simulink library "sp_lib"  (R2019a)
settings: Solver=VariableStepAuto  StartTime=0.0  StopTime=10.0  RelTol=1e-3
undefined symbols (not defined in the file or in its folder): collar_thick, diffuse, flange_len, flange_sep, flange_thick, flange_width, hex_rad, hex_skew, kind_val, leg_rad, lengths, lower_leg_len, shininess, specular, upper_leg_len, X, Y, Z
libraries: sm_lib x26, sm_stewart_platform_lib x10, nesl_utility x7
(part 1 of 2)
settings Model: Creator=mojo  LastModifiedBy=mojo

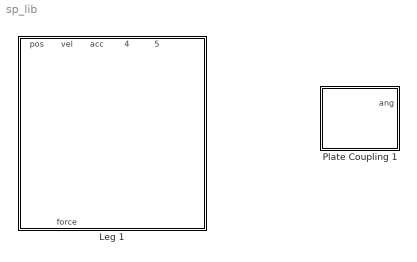
== system sp_lib ==
  Leg 1 : Subsystem  mask(Leg){upper_leg_len=upper_leg_len, lower_leg_len=lower_leg_len, rad=leg_rad, collar_thick=collar_thick, flange_len=flange_len, flange_width=flange_width, flange_thick=flange_thick, asm_offset=lengths(1)}
      mask prompts: upper_leg_len "Upper Leg Length (cm)"; lower_leg_len "Lower Leg Length (cm)"; rad "Radius (cm)"; collar_thick "Collar Thickness (cm)"; flange_len "Flange Length (cm)"; flange_width "Flange Width (cm)"; flange_thick "Flange Thickness (cm)"; asm_offset "Assembly Offset (cm)"
      mask help:
      | Models one of the six identical legs of a Stewart platform manipulator.
      |
      | Each leg is attached to two couplings: one on the base plate of the manipulator and a corresponding one on the platform plate of the manipulator.
      mask Help:
      | A <em>Leg</em> models one of the six identical legs of a Stewart platform manipulator.
      | 
      | Each leg is attached to two couplings: one on the base plate of the manipulator
      | and a corresponding one on the platform plate of the manipulator.
      | 
      | <h3>Components</h3>
      | 
      | A leg is an articulated, non-rigid structure comprising the following parts, listed in
      | top-to-bottom order in the typical orientation of the manipulator.
      | 
      | <ul>
      | <li> Shoulder crosspiece
      | <li> Revolute joint
      | <li> Upper leg
      | <li> Cylindrical knee joint
      | <li> Lower leg
      | <li> Revolute joint
      | <li> Ankle crosspiece
      | </ul>
      | 
      | The two revolute joints adjacent to the two crosspieces each form one half of a universal joint.  The other halves are modeled by revolute joints in the couplings to which the leg is connected.  These connections between legs and couplings could also be modeled by Universal Joint blocks, however, modeling these universal joints with pairs of revolute joints allows for a more detailed model that can display the motion of the universal joint crosspieces.
      | 
      | The leg is divided into upper and lower segments connected through a cylindrical knee joint.  The main portion of each of the two leg segments is modeled as a leg shaft.  Both segments have couplings attached; the upper leg also has a cylindrical extender bar attached.
      | 
      | The revolute primitive of the knee joint is completely passive; it is not actuated.  It is also not sensed.  However, the degree of freedom provided by this primitive is necessary to allow the Stewart platform to move.
      | 
      | The prismatic primitive of the knee joint is force actuated.  The force to be applied to this primitive is provided through a Simulink signal input. This primitive is also sensed: its (linear) position and velocity are available as two Simulink signal outputs.  Typically, a control system will read the current position and velocity and use these to determine a force to be applied to the prismatic primitive of the knee joint to achieve a desired motion of the platform.
      | 
      | Under normal operation, the position of the prismatic primitive of the knee joint should lie within the range [0, L], where L is the length of the lower leg segment.  In the zero configuration of the joint, the upper leg just touches the lower leg, with no gap between them.  A negative joint position will cause the two leg segments to intersect.  Positions exceeding L will cause the extender bar to completely leave the lower leg segment.
      | 
      | <h3>Leg Geometry</h3>
      | 
      | The <em>Geom</em> tab parameters specify the geometry of the main parts of the leg.
      | 
      | <ul>
      | 
      | <li> <b>Upper Leg Length</b> The length of the upper segment of the leg, including the thicknesses of the hexagonal collars but excluding the coupling and extender bar.
      | 
      | <li> <b>Lower Leg Length</b> The length of the lower segment of the leg, including the thicknesses of the hexagonal collars but excluding the coupling.
      | 
      | <li> <b>Radius</b> The radius of the hexagonal cross section of the upper and lower leg segments.
      | 
      | <li> <b>Collar Thickness</b> The thicknesses of the hexagonal collars the upper and lower leg segments.
      | 
      | </ul>
      | 
      | <h3>Flanges</h3>
      | 
      | The <em>Flanges</em> tab parameters specify the geometry of the flanges of the
      | couplings attached to the upper and lower legs.
      | 
      | <ul>
      | 
      | <li> <b>Flange Length</b> The length of the coupling flanges. See <em>Coupling</em> block for details.
      | 
      | <li> <b>Flange Width</b> The width of the coupling flanges. See <em>Coupling</em> block for details.
      | 
      | <li> <b>Flange Thickness</b> The thickness of the coupling flanges. See <em>Coupling</em> block for details.
      | 
      | </ul>
      | 
      | <h3>Assembly</h3>
      | 
      | The <em>Assembly</em> tab parameters specify values to be used during assembly of the Stewart Platform manipulator.
      | 
      | <ul>
      | 
      | <li><b>Assembly Offset</b> The estimated position of the prismatic primitive of the knee joint in the assembled configuration of the Stewart platform manipulator.  This value is used as a suggested joint target for the primitive; it does not have to be exact, and it may not be achieved exactly. Nonetheless, reasonable guesses of this value increase the chances of successful assembly of the manipulator.
      | 
      | </ul>
      | 
      | 
      | <h3>Visualization</h3>
      | 
      | The material properties of a leg's components are all pre-defined and not configurable.
      | 
      | <h3>Ports</h3>
      | 
      | <ul>
      | 
      | <li> <b>base</b> The frame on the leg that should be attached to a coupling on the manipulator's base plate.  This frame is attached to the ankle crosspiece.
      | 
      | <li> <b>platform</b> The frame on the leg that should be attached to a coupling on the manipulator's platform plate.  This frame is attached to the shoulder crosspiece.
      | 
      | <li><b>pos</b> The linear position of the prismatic primitive of the leg's knee joint as a Simulink signal output.  This signal is typically an input to a controller.
      | 
      | <li><b>vel</b> The linear velocity of the prismatic primitive of the leg's knee joint as a Simulink signal output.  This signal is typically an input to a controller.
      | 
      | <li><b>force</b> The force (in N) to be applied to the prismatic primitive of the leg's knee joint as a Simulink signal input.  This signal is typically specified by an output of a controller.  A positive force tends to increase the primitive position.
      | 
      | </ul>
      mask DialogControl ParameterTabVar0 Prompt: Geom
      mask DialogControl ParameterTabVar01 Prompt: Flanges
      mask DialogControl ParameterTabVar012 Prompt: Assembly
      mask Display:
      | image(imread('sm_stewart_platform_leg.png'))
      | color('white')
      | port_label('LConn', 1, 'base')
      | port_label('RConn', 1, 'platform')
      | color('yellow')
      | port_label('Input', 1, 'force')
      | port_label('Output', 1, 'pos')
      | port_label('Output', 2, 'vel')
      | port_label('Output', 3, 'acc')
      | port_label('Output', 4, 'base_ang')
      | port_label('Output', 5, 'plat_ang')
  Plate Coupling 1 : Subsystem  AncestorBlock=sm_stewart_platform_lib/Plate Coupling  mask(Plate Coupling){index=0 + kind_val, hex_rad=hex_rad, hex_skew=hex_skew, flange_width=flange_width, flange_thick=flange_thick, flange_sep=flange_sep, flange_ref_rot=kind_val * 180}
      mask prompts: index "Index (1-6)"; hex_rad "Hexagon Radius (cm)"; hex_skew "Hexagon Skew"; flange_width "Flange Width (cm)"; flange_thick "Flange Thickness (cm)"; flange_sep "Flange Separation (cm)"; flange_ref_rot "Flange Reference Rotation (deg)"
      mask help: Models a coupling with a rigid transform that places it in a specific position and orientation relative to a hexagon plate.
      mask init:
      | % index is in the range [0, 6)
      | sgn = 2 * mod(index + 1, 2) - 1;  % Alternating: +1, -1
      | alpha = (floor((index + 1) / 2) * 120  - 30) * pi/180;
      | theta = (index + sgn * hex_skew) * pi/3;
      | offset = [hex_rad, -(flange_sep + flange_thick) / 2, -flange_width / 2 * sgn] * ...
      |     [0 -sin(theta) +cos(theta); 0 -sin(alpha) +cos(alpha); 0 -cos(alpha) -sin(alpha)];
      mask Help:
      | A <em>Plate Coupling</em> models a coupling with a rigid transform that places it in a specific position and orientation relative to a hexagon plate.
      | 
      | This block serves a specialized role in the modeling of Stewart platform manipulator.  It is used to define the six couplings attached to the lower (base) and upper (platform) hexagon plates of the manipulator.  The plate coupling's initialization function performs the math needed to compute the proper rigid transforms.
      | 
      | <h3>Index</h3>
      | 
      | The <em>Index</em> tab parameters specify the index of the plate coupling.
      | 
      | <ul>
      | 
      | <li> <b>Index</b> The index of the plate coupling, which is an integer in the range [1, 6].  This value indicates which of the six couplings of a hexagonal plate is being defined.  It determines the parameters of the internal rigid transforms that place the coupling at one of the six corners of the skewed hexagon in the proper orientation.
      | 
      | </ul>
      | 
      | <h3>Geometry</h3>
      | 
      | The <em>Geom</em> tab parameters specify the geometry of the plate coupling.
      | 
      | <ul>
      | 
      | <li> <b>Hexagon Radius</b> The radius of the hexagon plate that this plate coupling is attached to.  See <em>Hexagon Plate</em> block for details.
      | 
      | <li> <b>Hexagon Skew</b> The skew factor of the hexagon plate that this plate coupling is attached to.  See <em>Hexagon Plate</em> block for details.
      | 
      | <li> <b>Flange Width</b> The width of the coupling flanges. See <em>Coupling</em> block for details.
      | 
      | <li> <b>Flange Thickness</b> The thickness of the coupling flanges. See <em>Coupling</em> block for details.
      | 
      | <li> <b>Flange Separation</b> The flange separation of the coupling. See <em>Coupling</em> block for details.
      | 
      | <li> <b>Flange Reference Rotation</b> The reference rotation of the coupling.  This value is set to zero for plate couplings attached to the top face of the base plate of the Stewart platform and to 180 degrees for plate couplings attached to the underside of the platform plate.  This aligns the x-axes of all couplings in the upward direction in the zero configuration. See <em>Coupling</em> for details.
      | 
      | </ul>
      | 
      | <h3>Ports</h3>
      | 
      | <ul>
      | 
      | <li> <b>plate</b> The frame of the plate coupling that should be rigidly attached to a frame in the center of the hexagon plate.  The z-axis of this latter frame should be oriented normal to the plane of the plate, and the z-coordinate of its origin should be in the plane of the universal joints attached to the plate.
      | 
      | <li> <b>leg</b> The frame of the plate coupling that should be attached to a leg of the Stewart platform.  Specifically, one of the two crosspieces of the leg is attached to this frame.  The other crosspiece is attached to a corresponding coupling on the other hexagon plate of the manipulator.
      | 
      | </ul>
      mask Display:
      | image(imread('sm_stewart_platform_platecoupling.png'))
      | port_label('LConn', 1, 'plate')
      | port_label('RConn', 1, 'leg')

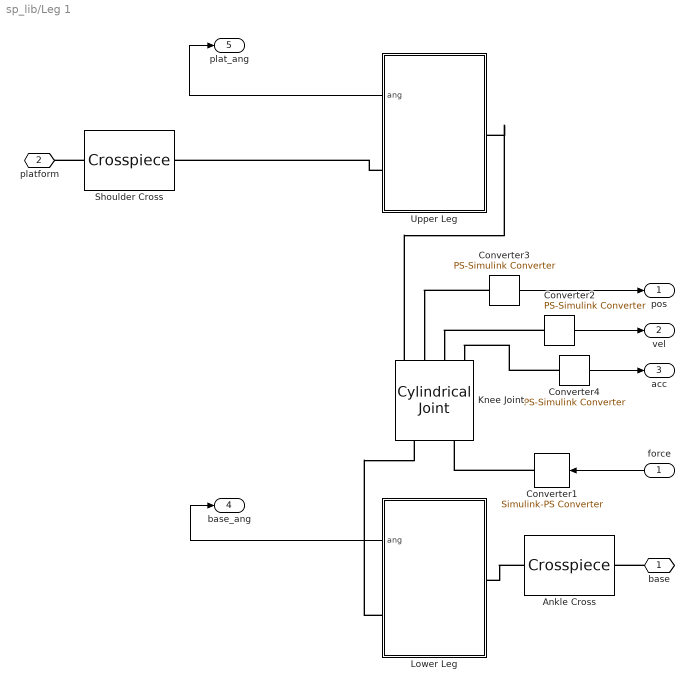
== system sp_lib/Leg 1 ==
  force : Inport
  Ankle Cross : sm_stewart_platform_lib/Crosspiece  arm_len=(rad - flange_thick) * 1.9  arm_rad=rad / 8.0
      settings: SourceProductName=Simscape Multibody  SourceProductBaseCode=MS
  Converter1 : nesl_utility/Simulink-PS Converter  PhysicalDomain=network_engine_domain  SubClassName=ps_input  LeftPortType=input  RightPortType=output  PseudoPeriodic=off  Frequencies=[]  NoiseDistribution=none  NoiseParameters=[]  Unit=N  AffineConversion=off  FilteringAndDerivatives=zero  SimscapeFilterOrder=1  InputFilterTimeConstant=.001  UdotUserProvided=0
  Converter2 : nesl_utility/PS-Simulink Converter  PhysicalDomain=network_engine_domain  SubClassName=ps_output  LeftPortType=input  RightPortType=output  PseudoPeriodic=off  Frequencies=[]  Unit=cm/s  AffineConversion=off
  Converter3 : nesl_utility/PS-Simulink Converter  PhysicalDomain=network_engine_domain  SubClassName=ps_output  LeftPortType=input  RightPortType=output  PseudoPeriodic=off  Frequencies=[]  Unit=cm  AffineConversion=off
  Converter4 : nesl_utility/PS-Simulink Converter  PhysicalDomain=network_engine_domain  SubClassName=ps_output  LeftPortType=input  RightPortType=output  PseudoPeriodic=off  Frequencies=[]  Unit=cm/s/s  AffineConversion=off
  Knee Joint : sm_lib/Joints/Cylindrical Joint  SenseConstraintForce=off  SenseConstraintForceX=off  SenseConstraintForceY=off  SenseConstraintForceZ=off  SenseConstraintTorque=off  SenseConstraintTorqueX=off  SenseConstraintTorqueY=off  SenseConstraintTorqueZ=off  SenseTotalForce=off  SenseTotalForceX=off  SenseTotalForceY=off  SenseTotalForceZ=off  SenseTotalTorque=off  SenseTotalTorqueX=off  SenseTotalTorqueY=off  SenseTotalTorqueZ=off  CompositeWrenchDir=FollowerOnBase  CompositeWrenchFrame=BaseFrame  PzEquilibriumPosition=0  PzEquilibriumPositionUnits=m  PzSpringStiffness=0  PzSpringStiffnessUnits=N/m  PzDampingCoefficient=0  PzDampingCoefficientUnits=N/(m/s)  PzTorqueActuationMode=InputTorque  PzMotionActuationMode=ComputedMotion  PzSensePosition=on  PzSenseVelocity=on  PzSenseAcceleration=on  PzSenseTorqueForce=off  PzSenseLowerLimitTorqueForce=off  PzSenseUpperLimitTorqueForce=off  PzLowerLimitSpecify=off  PzLowerLimitBound=-1  PzLowerLimitBoundUnits=m  PzLowerLimitStiffness=1e6  PzLowerLimitStiffnessUnits=N/m  PzLowerLimitDamping=1e3  PzLowerLimitDampingUnits=N/(m/s)  PzLowerLimitTransitionRegionWidth=1e-4  PzLowerLimitTransitionRegionWidthUnits=m  PzUpperLimitSpecify=off  PzUpperLimitBound=1  PzUpperLimitBoundUnits=m  PzUpperLimitStiffness=1e6  PzUpperLimitStiffnessUnits=N/m  PzUpperLimitDamping=1e3  PzUpperLimitDampingUnits=N/(m/s)  PzUpperLimitTransitionRegionWidth=1e-4  PzUpperLimitTransitionRegionWidthUnits=m  PzPositionTargetSpecify=on  PzPositionTargetPriority=High  PzPositionTargetValue=asm_offset  PzPositionTargetValueUnits=cm  PzVelocityTargetSpecify=off  PzVelocityTargetPriority=High  PzVelocityTargetValue=0  PzVelocityTargetValueUnits=m/s  RzEquilibriumPosition=0  RzEquilibriumPositionUnits=rad  RzSpringStiffness=0  RzSpringStiffnessUnits=N*m/rad  RzDampingCoefficient=0  RzDampingCoefficientUnits=N*m/(rad/s)  RzTorqueActuationMode=NoTorque  RzMotionActuationMode=ComputedMotion  RzSensePosition=off  RzSenseVelocity=off  RzSenseAcceleration=off  RzSenseTorqueForce=off  RzSenseLowerLimitTorqueForce=off  RzSenseUpperLimitTorqueForce=off  RzLowerLimitSpecify=off  RzLowerLimitBound=-90  RzLowerLimitBoundUnits=deg  RzLowerLimitStiffness=1e4  RzLowerLimitStiffnessUnits=N*m/deg  RzLowerLimitDamping=10  RzLowerLimitDampingUnits=N*m/(deg/s)  RzLowerLimitTransitionRegionWidth=0.1  RzLowerLimitTransitionRegionWidthUnits=deg  RzUpperLimitSpecify=off  RzUpperLimitBound=90  RzUpperLimitBoundUnits=deg  RzUpperLimitStiffness=1e4  RzUpperLimitStiffnessUnits=N*m/deg  RzUpperLimitDamping=10  RzUpperLimitDampingUnits=N*m/(deg/s)  RzUpperLimitTransitionRegionWidth=0.1  RzUpperLimitTransitionRegionWidthUnits=deg  RzPositionTargetSpecify=off  RzPositionTargetPriority=High  RzPositionTargetValue=0  RzPositionTargetValueUnits=rad  RzVelocityTargetSpecify=off  RzVelocityTargetPriority=High  RzVelocityTargetValue=0  RzVelocityTargetValueUnits=rad/s
  Lower Leg : Subsystem
      mask Display:
      | image(imread('sm_stewart_platform_lowerleg.png'))
      | color('white')
      | port_label('LConn', 1, 'lower')
      | port_label('RConn', 1, 'upper')
      | port_label('Output', 1, 'ang')
  Shoulder Cross : sm_stewart_platform_lib/Crosspiece  arm_len=(rad - flange_thick) * 1.9  arm_rad=rad / 8.0
      settings: SourceProductName=Simscape Multibody  SourceProductBaseCode=MS
  Upper Leg : Subsystem
      mask Display:
      | image(imread('sm_stewart_platform_upperleg.png'))
      | color('white')
      | port_label('LConn', 1, 'lower')
      | port_label('RConn', 1, 'upper')
      | port_label('Output', 1, 'ang')
  base : PMIOPort  Side=Left
  platform : PMIOPort  Port=2  Side=Right
  pos : Outport
  vel : Outport  Port=2
  acc : Outport  Port=3
  base_ang : Outport  Port=4
  plat_ang : Outport  Port=5
  wires:
  Converter3/1 -> pos/1
  Converter2/1 -> vel/1
  force/1 -> Converter1/1
  Converter4/1 -> acc/1
  Lower Leg/1(ang) -> base_ang/1
  Upper Leg/1(ang) -> plat_ang/1
  connections:
  Converter3/LConn1 -- Knee Joint/RConn2
  Converter2/LConn1 -- Knee Joint/RConn3
  Converter1/RConn1 -- Knee Joint/LConn2
  Knee Joint/RConn1 -- Upper Leg/LConn1
  Lower Leg/RConn1 -- Knee Joint/LConn1
  base/RConn1 -- Ankle Cross/LConn1
  Ankle Cross/RConn1 -- Lower Leg/LConn1
  Upper Leg/RConn1 -- Shoulder Cross/LConn1
  Shoulder Cross/RConn1 -- platform/RConn1
  Converter4/LConn1 -- Knee Joint/RConn4

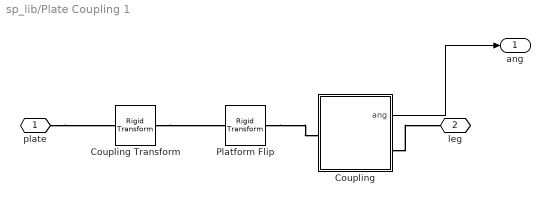
== system sp_lib/Plate Coupling 1 ==
  Coupling : Subsystem  AncestorBlock=sm_stewart_platform_lib/Coupling  mask(Coupling){flange_sep=flange_sep, flange_len=flange_len, flange_width=flange_width, flange_thick=flange_thick, ref_rot=flange_ref_rot, diffuse=diffuse, specular=specular, shininess=shininess}
      mask prompts: flange_sep "Flange Separation (cm)"; flange_len "Flange Length (cm)"; flange_width "Flange Width (cm)"; flange_thick "Flange Thickness (cm)"; ref_rot "Reference Rotation (deg)"; diffuse "Diffuse (rgba)"; specular "Specular (rgba)"; shininess "Shininess (0-128)"
      mask help: Models a pair of parallel flanges with a revolute joint between them.
      mask Help:
      | A <em>Coupling</em> models a pair of parallel flanges with a revolute joint between them.  The axis of the revolute joint is normal to the planes of the flanges.
      | 
      | In a Stewart platform, couplings attached to the base, legs, and platform are used to anchor the arms of the universal joint crosspieces.
      | 
      | <h3>Geometry</h3>
      | 
      | The <em>Geom</em> tab parameters specify the geometry of the coupling.
      | 
      | <ul>
      | 
      | <li> <b>Flange Separation</b> The distance between the origins of the reference frames of the two flanges.  These are located within the interiors of the flanges; the distance between the facing surfaces of the flanges is one flange thickness less than this amount.
      | 
      | <li> <b>Length</b> The length of the flanges.  See <em>Flange</em> block for details.
      | 
      | <li> <b>Width</b> The width of the flanges.  See <em>Flange</em> block for details.
      | 
      | <li> <b>Thickness</b> The thickness of the flanges.  See <em>Flange</em> block for details.
      | 
      | <li> <b>Reference Rotation</b> A value specifying the zero point for the coupling's revolute joint.  A value of zero makes the zero configuration the one in which the x-axis of the <em>rot</em> frame is directed toward the curved end caps of the flanges.  A value of 180 degrees makes the zero configuration the one in which the x-axis of the <em>rot</em> frame is directed away from the curved end caps of the flanges.
      | 
      | </ul>
      | 
      | <h3>Visualization</h3>
      | 
      | The <em>Graphics</em> tab parameters specify the visualization aspects of the coupling.  Both flanges of the coupling have the same visual properties.
      | 
      | <ul>
      | 
      | <li> <b>Diffuse</b> The diffuse color of the coupling.  This is an RGB 3-vector or an RGBA 4-vector with all components in the range [0, 1].
      | 
      | <li> <b>Specular</b> The specular color of the coupling.  This is an RGB 3-vector or an RGBA 4-vector with all components in the range [0, 1].
      | 
      | <li> <b>Shininess</b> The shininess of the coupling.  This is a scalar value in the range [0, 128].
      | 
      | </ul>
      | 
      | 
      | <h3>Ports</h3>
      | 
      | <ul>
      | 
      | <li> <b>ref</b> The reference frame of the coupling.  This is also the base frame of the coupling's revolute joint.  The origin is at the midpoint of the line segment joining the reference frame origins of the two flanges.  The z-axis is normal to the planes of the flanges.  The x-axis direction depends on the setting of <em>Reference Roation</em> (see above).
      | 
      | <li> <b>rot</b> The rotated frame of the coupling.  This is also the follower frame of the coupling's revolute joint.  The origin is at the midpoint of the line segment joining the reference frame origins of the two flanges.  The z-axis is normal to the planes of the flanges.  The x-axis direction depends on the setting of <em>Reference Roation</em> (see above) and on the revolute joint's position.
      | 
      | </ul>
      | 
      | Typically, a coupling is rigidly attached to a host body through its <em>ref</em> port.  The body attached to its <em>rot</em> port can rotate about the coupling axis with respect to the host body.
      mask Display:
      | image(imread('sm_stewart_platform_coupling.png'))
      | color('white')
      | port_label('LConn', 1, 'ref')
      | port_label('RConn', 1, 'rot')
  Coupling Transform : sm_lib/Frames and Transforms/Rigid Transform  TranslationMethod=Cartesian  TranslationStandardOffset=0  TranslationLengthUnit=cm  TranslationStandardAxis=+Z  TranslationCartesianOffset=offset  TranslationROffset=0  TranslationROffsetUnits=m  TranslationZOffset=0  TranslationZOffsetUnits=m  TranslationThetaOffset=0  TranslationThetaOffsetUnits=deg  RotationMethod=StandardAxis  RotationAngleUnits=rad  RotationStandardAxis=+X  RotationAngle=alpha  RotationArbitraryAxis=[0 0 1]  FollAlignAxisA=+X  BaseAlignAxisA=+Y  FollAlignAxisB=+Y  BaseAlignAxisB=+Z  RotationSequenceAxes=FollowerAxes  RotationSequence=XYX  RotationSequenceAngles=[0 0 0]  RotationSequenceAnglesUnits=deg  RotationMatrix=[1 0 0; 0 1 0; 0 0 1]
  Platform Flip : sm_lib/Frames and Transforms/Rigid Transform  TranslationMethod=None  TranslationStandardOffset=0  TranslationLengthUnit=m  TranslationStandardAxis=+Z  TranslationCartesianOffset=[0 0 0]  TranslationROffset=0  TranslationROffsetUnits=m  TranslationZOffset=0  TranslationZOffsetUnits=m  TranslationThetaOffset=0  TranslationThetaOffsetUnits=deg  RotationMethod=StandardAxis  RotationAngleUnits=deg  RotationStandardAxis=+Z  RotationAngle=kind_val * 180  RotationArbitraryAxis=[0 0 1]  FollAlignAxisA=+X  BaseAlignAxisA=+Y  FollAlignAxisB=+Y  BaseAlignAxisB=+Z  RotationSequenceAxes=FollowerAxes  RotationSequence=XYX  RotationSequenceAngles=[0 0 0]  RotationSequenceAnglesUnits=deg  RotationMatrix=[1 0 0; 0 1 0; 0 0 1]
  plate : PMIOPort  Side=Left
  leg : PMIOPort  Port=2  Side=Right
  ang : Outport
  wires:
  Coupling/1(ang) -> ang/1
  connections:
  plate/RConn1 -- Coupling Transform/LConn1
  Coupling Transform/RConn1 -- Platform Flip/LConn1
  Platform Flip/RConn1 -- Coupling/LConn1
  Coupling/RConn1 -- leg/RConn1

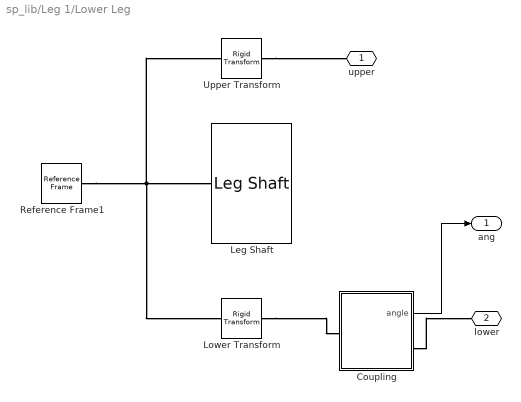
== system sp_lib/Leg 1/Lower Leg ==
  Coupling : Subsystem  AncestorBlock=sm_stewart_platform_lib/Coupling  mask(Coupling){flange_sep=2 * rad * cos(pi/6) - flange_thick, flange_len=flange_len, flange_width=flange_width, flange_thick=flange_thick, ref_rot=180, diffuse=[.5 .5 .6], specular=[.8 .8 1], shininess=100}
      mask prompts: flange_sep "Flange Separation (cm)"; flange_len "Flange Length (cm)"; flange_width "Flange Width (cm)"; flange_thick "Flange Thickness (cm)"; ref_rot "Reference Rotation (deg)"; diffuse "Diffuse (rgba)"; specular "Specular (rgba)"; shininess "Shininess (0-128)"
      mask help: Models a pair of parallel flanges with a revolute joint between them.
      mask Help:
      | A <em>Coupling</em> models a pair of parallel flanges with a revolute joint between them.  The axis of the revolute joint is normal to the planes of the flanges.
      | 
      | In a Stewart platform, couplings attached to the base, legs, and platform are used to anchor the arms of the universal joint crosspieces.
      | 
      | <h3>Geometry</h3>
      | 
      | The <em>Geom</em> tab parameters specify the geometry of the coupling.
      | 
      | <ul>
      | 
      | <li> <b>Flange Separation</b> The distance between the origins of the reference frames of the two flanges.  These are located within the interiors of the flanges; the distance between the facing surfaces of the flanges is one flange thickness less than this amount.
      | 
      | <li> <b>Length</b> The length of the flanges.  See <em>Flange</em> block for details.
      | 
      | <li> <b>Width</b> The width of the flanges.  See <em>Flange</em> block for details.
      | 
      | <li> <b>Thickness</b> The thickness of the flanges.  See <em>Flange</em> block for details.
      | 
      | <li> <b>Reference Rotation</b> A value specifying the zero point for the coupling's revolute joint.  A value of zero makes the zero configuration the one in which the x-axis of the <em>rot</em> frame is directed toward the curved end caps of the flanges.  A value of 180 degrees makes the zero configuration the one in which the x-axis of the <em>rot</em> frame is directed away from the curved end caps of the flanges.
      | 
      | </ul>
      | 
      | <h3>Visualization</h3>
      | 
      | The <em>Graphics</em> tab parameters specify the visualization aspects of the coupling.  Both flanges of the coupling have the same visual properties.
      | 
      | <ul>
      | 
      | <li> <b>Diffuse</b> The diffuse color of the coupling.  This is an RGB 3-vector or an RGBA 4-vector with all components in the range [0, 1].
      | 
      | <li> <b>Specular</b> The specular color of the coupling.  This is an RGB 3-vector or an RGBA 4-vector with all components in the range [0, 1].
      | 
      | <li> <b>Shininess</b> The shininess of the coupling.  This is a scalar value in the range [0, 128].
      | 
      | </ul>
      | 
      | 
      | <h3>Ports</h3>
      | 
      | <ul>
      | 
      | <li> <b>ref</b> The reference frame of the coupling.  This is also the base frame of the coupling's revolute joint.  The origin is at the midpoint of the line segment joining the reference frame origins of the two flanges.  The z-axis is normal to the planes of the flanges.  The x-axis direction depends on the setting of <em>Reference Roation</em> (see above).
      | 
      | <li> <b>rot</b> The rotated frame of the coupling.  This is also the follower frame of the coupling's revolute joint.  The origin is at the midpoint of the line segment joining the reference frame origins of the two flanges.  The z-axis is normal to the planes of the flanges.  The x-axis direction depends on the setting of <em>Reference Roation</em> (see above) and on the revolute joint's position.
      | 
      | </ul>
      | 
      | Typically, a coupling is rigidly attached to a host body through its <em>ref</em> port.  The body attached to its <em>rot</em> port can rotate about the coupling axis with respect to the host body.
      mask Display:
      | image(imread('sm_stewart_platform_coupling.png'))
      | color('white')
      | port_label('LConn', 1, 'ref')
      | port_label('RConn', 1, 'rot')
  Leg Shaft : sm_stewart_platform_lib/Leg Shaft  length=lower_leg_len  rad=rad  collar_thick=collar_thick  color=[0 0 0.6]
      settings: SourceProductName=Simscape Multibody  SourceProductBaseCode=MS
  Lower Transform : sm_lib/Frames and Transforms/Rigid Transform  TranslationMethod=StandardAxis  TranslationStandardOffset=lower_leg_len / 2 + flange_len  TranslationLengthUnit=cm  TranslationStandardAxis=-Z  TranslationCartesianOffset=[0 0 0]  TranslationROffset=0  TranslationROffsetUnits=m  TranslationZOffset=0  TranslationZOffsetUnits=m  TranslationThetaOffset=0  TranslationThetaOffsetUnits=deg  RotationMethod=AlignedAxes  RotationAngleUnits=deg  RotationStandardAxis=+Z  RotationAngle=0  RotationArbitraryAxis=[0 0 1]  FollAlignAxisA=+Z  BaseAlignAxisA=+X  FollAlignAxisB=+X  BaseAlignAxisB=-Z  RotationSequenceAxes=FollowerAxes  RotationSequence=XYX  RotationSequenceAngles=[0 0 0]  RotationSequenceAnglesUnits=deg  RotationMatrix=[1 0 0; 0 1 0; 0 0 1]
  Reference Frame1 : sm_lib/Frames and Transforms/Reference Frame
  Upper Transform : sm_lib/Frames and Transforms/Rigid Transform  TranslationMethod=StandardAxis  TranslationStandardOffset=lower_leg_len / 2  TranslationLengthUnit=cm  TranslationStandardAxis=+Z  TranslationCartesianOffset=[0 0 0]  TranslationROffset=0  TranslationROffsetUnits=m  TranslationZOffset=0  TranslationZOffsetUnits=m  TranslationThetaOffset=0  TranslationThetaOffsetUnits=deg  RotationMethod=None  RotationAngleUnits=deg  RotationStandardAxis=+Z  RotationAngle=0  RotationArbitraryAxis=[0 0 1]  FollAlignAxisA=+X  BaseAlignAxisA=+Y  FollAlignAxisB=+Y  BaseAlignAxisB=+Z  RotationSequenceAxes=FollowerAxes  RotationSequence=XYX  RotationSequenceAngles=[0 0 0]  RotationSequenceAnglesUnits=deg  RotationMatrix=[1 0 0; 0 1 0; 0 0 1]
  upper : PMIOPort  Side=Right
  lower : PMIOPort  Port=2  Side=Left
  ang : Outport
  wires:
  Coupling/1(angle) -> ang/1
  connections:
  Reference Frame1/RConn1 -- Upper Transform/LConn1 -- Lower Transform/LConn1 -- Leg Shaft/LConn1
  Coupling/RConn1 -- lower/RConn1
  Upper Transform/RConn1 -- upper/RConn1
  Lower Transform/RConn1 -- Coupling/LConn1

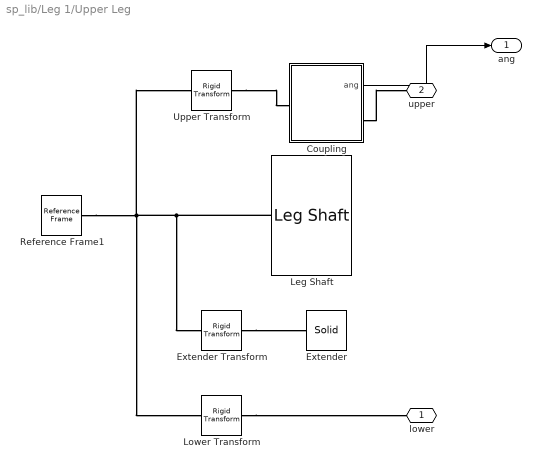
== system sp_lib/Leg 1/Upper Leg ==
  Coupling : Subsystem  AncestorBlock=sm_stewart_platform_lib/Coupling  mask(Coupling){flange_sep=2 * rad * cos(pi/6) - flange_thick, flange_len=flange_len, flange_width=flange_width, flange_thick=flange_thick, ref_rot=0, diffuse=[.5 .5 .6], specular=[.8 .8 1], shininess=100}
      mask prompts: flange_sep "Flange Separation (cm)"; flange_len "Flange Length (cm)"; flange_width "Flange Width (cm)"; flange_thick "Flange Thickness (cm)"; ref_rot "Reference Rotation (deg)"; diffuse "Diffuse (rgba)"; specular "Specular (rgba)"; shininess "Shininess (0-128)"
      mask help: Models a pair of parallel flanges with a revolute joint between them.
      mask Help:
      | A <em>Coupling</em> models a pair of parallel flanges with a revolute joint between them.  The axis of the revolute joint is normal to the planes of the flanges.
      | 
      | In a Stewart platform, couplings attached to the base, legs, and platform are used to anchor the arms of the universal joint crosspieces.
      | 
      | <h3>Geometry</h3>
      | 
      | The <em>Geom</em> tab parameters specify the geometry of the coupling.
      | 
      | <ul>
      | 
      | <li> <b>Flange Separation</b> The distance between the origins of the reference frames of the two flanges.  These are located within the interiors of the flanges; the distance between the facing surfaces of the flanges is one flange thickness less than this amount.
      | 
      | <li> <b>Length</b> The length of the flanges.  See <em>Flange</em> block for details.
      | 
      | <li> <b>Width</b> The width of the flanges.  See <em>Flange</em> block for details.
      | 
      | <li> <b>Thickness</b> The thickness of the flanges.  See <em>Flange</em> block for details.
      | 
      | <li> <b>Reference Rotation</b> A value specifying the zero point for the coupling's revolute joint.  A value of zero makes the zero configuration the one in which the x-axis of the <em>rot</em> frame is directed toward the curved end caps of the flanges.  A value of 180 degrees makes the zero configuration the one in which the x-axis of the <em>rot</em> frame is directed away from the curved end caps of the flanges.
      | 
      | </ul>
      | 
      | <h3>Visualization</h3>
      | 
      | The <em>Graphics</em> tab parameters specify the visualization aspects of the coupling.  Both flanges of the coupling have the same visual properties.
      | 
      | <ul>
      | 
      | <li> <b>Diffuse</b> The diffuse color of the coupling.  This is an RGB 3-vector or an RGBA 4-vector with all components in the range [0, 1].
      | 
      | <li> <b>Specular</b> The specular color of the coupling.  This is an RGB 3-vector or an RGBA 4-vector with all components in the range [0, 1].
      | 
      | <li> <b>Shininess</b> The shininess of the coupling.  This is a scalar value in the range [0, 128].
      | 
      | </ul>
      | 
      | 
      | <h3>Ports</h3>
      | 
      | <ul>
      | 
      | <li> <b>ref</b> The reference frame of the coupling.  This is also the base frame of the coupling's revolute joint.  The origin is at the midpoint of the line segment joining the reference frame origins of the two flanges.  The z-axis is normal to the planes of the flanges.  The x-axis direction depends on the setting of <em>Reference Roation</em> (see above).
      | 
      | <li> <b>rot</b> The rotated frame of the coupling.  This is also the follower frame of the coupling's revolute joint.  The origin is at the midpoint of the line segment joining the reference frame origins of the two flanges.  The z-axis is normal to the planes of the flanges.  The x-axis direction depends on the setting of <em>Reference Roation</em> (see above) and on the revolute joint's position.
      | 
      | </ul>
      | 
      | Typically, a coupling is rigidly attached to a host body through its <em>ref</em> port.  The body attached to its <em>rot</em> port can rotate about the coupling axis with respect to the host body.
      mask Display:
      | image(imread('sm_stewart_platform_coupling.png'))
      | color('white')
      | port_label('LConn', 1, 'ref')
      | port_label('RConn', 1, 'rot')
  Extender : sm_lib/Body Elements/Solid  InertiaType=CalculateFromGeometry  Mass=1  MassUnits=kg  CenterOfMass=[0 0 0]  CenterOfMassUnits=m  MomentsOfInertia=[1 1 1]  MomentsOfInertiaUnits=kg*m^2  ProductsOfInertia=[0 0 0]  ProductsOfInertiaUnits=kg*m^2  BasedOnType=Density  Density=g_density  DensityUnits=g/cm^3  DoExposeReferenceFrame=on  SerializedFrames=<Frames/>  GraphicType=FromGeometry  MarkerShape=Sphere  MarkerSize=1  MarkerSizeUnits=m  GraphicVisPropType=AdvancedVisualProperties  GraphicDiffuseColor=[.5 .5 .6]  GraphicSpecularColor=[.8 .8 1]  GraphicAmbientColor=[ 0.1 0.1 0.1 ]  GraphicEmissiveColor=[ 0 0 0]  GraphicShininess=100  GraphicOpacity=1  GeometryShape=Cylinder  RectangleSize=[1 1]  RectangleSizeUnits=m  BrickDimensions=[1 1 1]  BrickDimensionUnits=m  CylinderRadius=rad / 2  CylinderRadiusUnits=cm  CylinderLength=lower_leg_len  CylinderLengthUnits=cm  SphereRadius=1  SphereRadiusUnits=m  EllipsoidRadii=[1 1 1]  EllipsoidRadiiUnits=m  ExtrusionCrossSection=[1 1; -1 1; -1 -1; 1 -1]  ExtrusionCrossSectionUnits=m  ExtrusionLength=lower_leg_len  ExtrusionLengthUnits=cm  PolygonNumSides=6  PolygonOuterRadius=rad / 2  PolygonOuterRadiusUnits=cm  ExtGeomFileType=STEP  ExtGeomFileUnits=m  RevolutionCrossSection=[1 1; 1 -1; 2 -1; 2 1]  RevolutionCrossSectionUnits=m  RevolutionExtent=Full  RevolutionAngle=180  RevolutionAngleUnits=deg
  Extender Transform : sm_lib/Frames and Transforms/Rigid Transform  TranslationMethod=StandardAxis  TranslationStandardOffset=(upper_leg_len + lower_leg_len) / 2  TranslationLengthUnit=cm  TranslationStandardAxis=-Z  TranslationCartesianOffset=[0 0 0]  TranslationROffset=0  TranslationROffsetUnits=m  TranslationZOffset=0  TranslationZOffsetUnits=m  TranslationThetaOffset=0  TranslationThetaOffsetUnits=deg  RotationMethod=StandardAxis  RotationAngleUnits=deg  RotationStandardAxis=+Z  RotationAngle=30  RotationArbitraryAxis=[0 0 1]  FollAlignAxisA=+X  BaseAlignAxisA=+Y  FollAlignAxisB=+Y  BaseAlignAxisB=+Z  RotationSequenceAxes=FollowerAxes  RotationSequence=XYX  RotationSequenceAngles=[0 0 0]  RotationSequenceAnglesUnits=deg  RotationMatrix=[1 0 0; 0 1 0; 0 0 1]
  Leg Shaft : sm_stewart_platform_lib/Leg Shaft  length=upper_leg_len  rad=rad  collar_thick=collar_thick  color=[0.6 0 0]
      settings: SourceProductName=Simscape Multibody  SourceProductBaseCode=MS
  Lower Transform : sm_lib/Frames and Transforms/Rigid Transform  TranslationMethod=StandardAxis  TranslationStandardOffset=upper_leg_len / 2  TranslationLengthUnit=cm  TranslationStandardAxis=-Z  TranslationCartesianOffset=[0 0 0]  TranslationROffset=0  TranslationROffsetUnits=m  TranslationZOffset=0  TranslationZOffsetUnits=m  TranslationThetaOffset=0  TranslationThetaOffsetUnits=deg  RotationMethod=None  RotationAngleUnits=deg  RotationStandardAxis=+Z  RotationAngle=0  RotationArbitraryAxis=[0 0 1]  FollAlignAxisA=+X  BaseAlignAxisA=+Y  FollAlignAxisB=+Y  BaseAlignAxisB=+Z  RotationSequenceAxes=FollowerAxes  RotationSequence=XYX  RotationSequenceAngles=[0 0 0]  RotationSequenceAnglesUnits=deg  RotationMatrix=[1 0 0; 0 1 0; 0 0 1]
  Reference Frame1 : sm_lib/Frames and Transforms/Reference Frame
  Upper Transform : sm_lib/Frames and Transforms/Rigid Transform  TranslationMethod=StandardAxis  TranslationStandardOffset=upper_leg_len / 2 + flange_len  TranslationLengthUnit=cm  TranslationStandardAxis=+Z  TranslationCartesianOffset=[0 0 0]  TranslationROffset=0  TranslationROffsetUnits=m  TranslationZOffset=0  TranslationZOffsetUnits=m  TranslationThetaOffset=0  TranslationThetaOffsetUnits=deg  RotationMethod=AlignedAxes  RotationAngleUnits=deg  RotationStandardAxis=+Z  RotationAngle=0  RotationArbitraryAxis=[0 0 1]  FollAlignAxisA=+Z  BaseAlignAxisA=-X  FollAlignAxisB=+X  BaseAlignAxisB=+Z  RotationSequenceAxes=FollowerAxes  RotationSequence=XYX  RotationSequenceAngles=[0 0 0]  RotationSequenceAnglesUnits=deg  RotationMatrix=[1 0 0; 0 1 0; 0 0 1]
  lower : PMIOPort  Side=Left
  upper : PMIOPort  Port=2  Side=Right
  ang : Outport
  wires:
  Coupling/1(ang) -> ang/1
  connections:
  Upper Transform/RConn1 -- Coupling/LConn1
  Lower Transform/RConn1 -- lower/RConn1
  Coupling/RConn1 -- upper/RConn1
  Leg Shaft/LConn1 -- Reference Frame1/RConn1 -- Upper Transform/LConn1 -- Lower Transform/LConn1 -- Extender Transform/LConn1
  Extender Transform/RConn1 -- Extender/RConn1

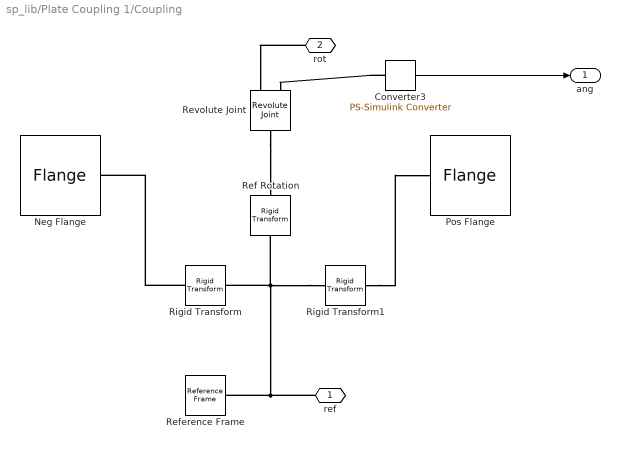
== system sp_lib/Plate Coupling 1/Coupling ==
  Converter3 : nesl_utility/PS-Simulink Converter  PhysicalDomain=network_engine_domain  SubClassName=ps_output  LeftPortType=input  RightPortType=output  PseudoPeriodic=off  Frequencies=[]  Unit=deg  AffineConversion=off
  Neg Flange : sm_stewart_platform_lib/Flange  len=flange_len  width=flange_width  thick=flange_thick  diffuse=diffuse  specular=specular  shininess=shininess
      settings: SourceProductName=Simscape Multibody  SourceProductBaseCode=MS
  Pos Flange : sm_stewart_platform_lib/Flange  len=flange_len  width=flange_width  thick=flange_thick  diffuse=diffuse  specular=specular  shininess=shininess
      settings: SourceProductName=Simscape Multibody  SourceProductBaseCode=MS
  Ref Rotation : sm_lib/Frames and Transforms/Rigid Transform  TranslationMethod=None  TranslationStandardOffset=0  TranslationLengthUnit=m  TranslationStandardAxis=+Z  TranslationCartesianOffset=[0 0 0]  TranslationROffset=0  TranslationROffsetUnits=m  TranslationZOffset=0  TranslationZOffsetUnits=m  TranslationThetaOffset=0  TranslationThetaOffsetUnits=deg  RotationMethod=StandardAxis  RotationAngleUnits=deg  RotationStandardAxis=+Z  RotationAngle=ref_rot  RotationArbitraryAxis=[0 0 1]  FollAlignAxisA=+X  BaseAlignAxisA=+Y  FollAlignAxisB=+Y  BaseAlignAxisB=+Z  RotationSequenceAxes=FollowerAxes  RotationSequence=XYX  RotationSequenceAngles=[0 0 0]  RotationSequenceAnglesUnits=deg  RotationMatrix=[1 0 0; 0 1 0; 0 0 1]
  Reference Frame : sm_lib/Frames and Transforms/Reference Frame
  Revolute Joint : sm_lib/Joints/Revolute Joint  SenseConstraintForce=off  SenseConstraintForceX=off  SenseConstraintForceY=off  SenseConstraintForceZ=off  SenseConstraintTorque=off  SenseConstraintTorqueX=off  SenseConstraintTorqueY=off  SenseConstraintTorqueZ=off  SenseTotalForce=off  SenseTotalForceX=off  SenseTotalForceY=off  SenseTotalForceZ=off  SenseTotalTorque=off  SenseTotalTorqueX=off  SenseTotalTorqueY=off  SenseTotalTorqueZ=off  CompositeWrenchDir=FollowerOnBase  CompositeWrenchFrame=BaseFrame  EquilibriumPosition=0  EquilibriumPositionUnits=rad  SpringStiffness=0  SpringStiffnessUnits=N*m/rad  DampingCoefficient=0  DampingCoefficientUnits=N*m/(rad/s)  TorqueActuationMode=NoTorque  MotionActuationMode=ComputedMotion  SensePosition=on  SenseVelocity=off  SenseAcceleration=off  SenseTorqueForce=off  SenseLowerLimitTorqueForce=off  SenseUpperLimitTorqueForce=off  LowerLimitSpecify=off  LowerLimitBound=-90  LowerLimitBoundUnits=deg  LowerLimitStiffness=1e4  LowerLimitStiffnessUnits=N*m/deg  LowerLimitDamping=10  LowerLimitDampingUnits=N*m/(deg/s)  LowerLimitTransitionRegionWidth=0.1  LowerLimitTransitionRegionWidthUnits=deg  UpperLimitSpecify=off  UpperLimitBound=90  UpperLimitBoundUnits=deg  UpperLimitStiffness=1e4  UpperLimitStiffnessUnits=N*m/deg  UpperLimitDamping=10  UpperLimitDampingUnits=N*m/(deg/s)  UpperLimitTransitionRegionWidth=0.1  UpperLimitTransitionRegionWidthUnits=deg  PositionTargetSpecify=off  PositionTargetPriority=High  PositionTargetValue=0  PositionTargetValueUnits=rad  VelocityTargetSpecify=off  VelocityTargetPriority=High  VelocityTargetValue=0  VelocityTargetValueUnits=rad/s
  Rigid Transform : sm_lib/Frames and Transforms/Rigid Transform  TranslationMethod=StandardAxis  TranslationStandardOffset=flange_sep / 2  TranslationLengthUnit=cm  TranslationStandardAxis=-Z  TranslationCartesianOffset=[0 0 0]  TranslationROffset=0  TranslationROffsetUnits=m  TranslationZOffset=0  TranslationZOffsetUnits=m  TranslationThetaOffset=0  TranslationThetaOffsetUnits=deg  RotationMethod=None  RotationAngleUnits=deg  RotationStandardAxis=+Z  RotationAngle=0  RotationArbitraryAxis=[0 0 1]  FollAlignAxisA=+X  BaseAlignAxisA=+Y  FollAlignAxisB=+Y  BaseAlignAxisB=+Z  RotationSequenceAxes=FollowerAxes  RotationSequence=XYX  RotationSequenceAngles=[0 0 0]  RotationSequenceAnglesUnits=deg  RotationMatrix=[1 0 0; 0 1 0; 0 0 1]
  Rigid Transform1 : sm_lib/Frames and Transforms/Rigid Transform  TranslationMethod=StandardAxis  TranslationStandardOffset=flange_sep / 2  TranslationLengthUnit=cm  TranslationStandardAxis=+Z  TranslationCartesianOffset=[0 0 0]  TranslationROffset=0  TranslationROffsetUnits=m  TranslationZOffset=0  TranslationZOffsetUnits=m  TranslationThetaOffset=0  TranslationThetaOffsetUnits=deg  RotationMethod=None  RotationAngleUnits=deg  RotationStandardAxis=+Z  RotationAngle=0  RotationArbitraryAxis=[0 0 1]  FollAlignAxisA=+X  BaseAlignAxisA=+Y  FollAlignAxisB=+Y  BaseAlignAxisB=+Z  RotationSequenceAxes=FollowerAxes  RotationSequence=XYX  RotationSequenceAngles=[0 0 0]  RotationSequenceAnglesUnits=deg  RotationMatrix=[1 0 0; 0 1 0; 0 0 1]
  ref : PMIOPort  Side=Left
  rot : PMIOPort  Port=2  Side=Right
  ang : Outport
  wires:
  Converter3/1 -> ang/1
  connections:
  Converter3/LConn1 -- Revolute Joint/RConn2
  Rigid Transform1/LConn1 -- Rigid Transform/LConn1 -- Ref Rotation/LConn1 -- Reference Frame/RConn1 -- ref/RConn1
  Rigid Transform/RConn1 -- Neg Flange/RConn1
  Rigid Transform1/RConn1 -- Pos Flange/RConn1
  rot/RConn1 -- Revolute Joint/RConn1
  Revolute Joint/LConn1 -- Ref Rotation/RConn1

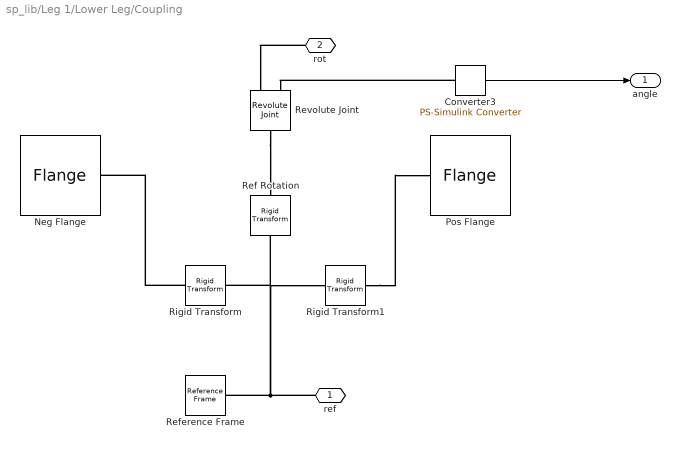
== system sp_lib/Leg 1/Lower Leg/Coupling ==
  Converter3 : nesl_utility/PS-Simulink Converter  PhysicalDomain=network_engine_domain  SubClassName=ps_output  LeftPortType=input  RightPortType=output  PseudoPeriodic=off  Frequencies=[]  Unit=deg  AffineConversion=off
  Neg Flange : sm_stewart_platform_lib/Flange  len=flange_len  width=flange_width  thick=flange_thick  diffuse=diffuse  specular=specular  shininess=shininess
      settings: SourceProductName=Simscape Multibody  SourceProductBaseCode=MS
  Pos Flange : sm_stewart_platform_lib/Flange  len=flange_len  width=flange_width  thick=flange_thick  diffuse=diffuse  specular=specular  shininess=shininess
      settings: SourceProductName=Simscape Multibody  SourceProductBaseCode=MS
  Ref Rotation : sm_lib/Frames and Transforms/Rigid Transform  TranslationMethod=None  TranslationStandardOffset=0  TranslationLengthUnit=m  TranslationStandardAxis=+Z  TranslationCartesianOffset=[0 0 0]  TranslationROffset=0  TranslationROffsetUnits=m  TranslationZOffset=0  TranslationZOffsetUnits=m  TranslationThetaOffset=0  TranslationThetaOffsetUnits=deg  RotationMethod=StandardAxis  RotationAngleUnits=deg  RotationStandardAxis=+Z  RotationAngle=ref_rot  RotationArbitraryAxis=[0 0 1]  FollAlignAxisA=+X  BaseAlignAxisA=+Y  FollAlignAxisB=+Y  BaseAlignAxisB=+Z  RotationSequenceAxes=FollowerAxes  RotationSequence=XYX  RotationSequenceAngles=[0 0 0]  RotationSequenceAnglesUnits=deg  RotationMatrix=[1 0 0; 0 1 0; 0 0 1]
  Reference Frame : sm_lib/Frames and Transforms/Reference Frame
  Revolute Joint : sm_lib/Joints/Revolute Joint  SenseConstraintForce=off  SenseConstraintForceX=off  SenseConstraintForceY=off  SenseConstraintForceZ=off  SenseConstraintTorque=off  SenseConstraintTorqueX=off  SenseConstraintTorqueY=off  SenseConstraintTorqueZ=off  SenseTotalForce=off  SenseTotalForceX=off  SenseTotalForceY=off  SenseTotalForceZ=off  SenseTotalTorque=off  SenseTotalTorqueX=off  SenseTotalTorqueY=off  SenseTotalTorqueZ=off  CompositeWrenchDir=FollowerOnBase  CompositeWrenchFrame=BaseFrame  EquilibriumPosition=0  EquilibriumPositionUnits=rad  SpringStiffness=0  SpringStiffnessUnits=N*m/rad  DampingCoefficient=0  DampingCoefficientUnits=N*m/(rad/s)  TorqueActuationMode=NoTorque  MotionActuationMode=ComputedMotion  SensePosition=on  SenseVelocity=off  SenseAcceleration=off  SenseTorqueForce=off  SenseLowerLimitTorqueForce=off  SenseUpperLimitTorqueForce=off  LowerLimitSpecify=off  LowerLimitBound=-90  LowerLimitBoundUnits=deg  LowerLimitStiffness=1e4  LowerLimitStiffnessUnits=N*m/deg  LowerLimitDamping=10  LowerLimitDampingUnits=N*m/(deg/s)  LowerLimitTransitionRegionWidth=0.1  LowerLimitTransitionRegionWidthUnits=deg  UpperLimitSpecify=off  UpperLimitBound=90  UpperLimitBoundUnits=deg  UpperLimitStiffness=1e4  UpperLimitStiffnessUnits=N*m/deg  UpperLimitDamping=10  UpperLimitDampingUnits=N*m/(deg/s)  UpperLimitTransitionRegionWidth=0.1  UpperLimitTransitionRegionWidthUnits=deg  PositionTargetSpecify=off  PositionTargetPriority=High  PositionTargetValue=0  PositionTargetValueUnits=rad  VelocityTargetSpecify=off  VelocityTargetPriority=High  VelocityTargetValue=0  VelocityTargetValueUnits=rad/s
  Rigid Transform : sm_lib/Frames and Transforms/Rigid Transform  TranslationMethod=StandardAxis  TranslationStandardOffset=flange_sep / 2  TranslationLengthUnit=cm  TranslationStandardAxis=-Z  TranslationCartesianOffset=[0 0 0]  TranslationROffset=0  TranslationROffsetUnits=m  TranslationZOffset=0  TranslationZOffsetUnits=m  TranslationThetaOffset=0  TranslationThetaOffsetUnits=deg  RotationMethod=None  RotationAngleUnits=deg  RotationStandardAxis=+Z  RotationAngle=0  RotationArbitraryAxis=[0 0 1]  FollAlignAxisA=+X  BaseAlignAxisA=+Y  FollAlignAxisB=+Y  BaseAlignAxisB=+Z  RotationSequenceAxes=FollowerAxes  RotationSequence=XYX  RotationSequenceAngles=[0 0 0]  RotationSequenceAnglesUnits=deg  RotationMatrix=[1 0 0; 0 1 0; 0 0 1]
  Rigid Transform1 : sm_lib/Frames and Transforms/Rigid Transform  TranslationMethod=StandardAxis  TranslationStandardOffset=flange_sep / 2  TranslationLengthUnit=cm  TranslationStandardAxis=+Z  TranslationCartesianOffset=[0 0 0]  TranslationROffset=0  TranslationROffsetUnits=m  TranslationZOffset=0  TranslationZOffsetUnits=m  TranslationThetaOffset=0  TranslationThetaOffsetUnits=deg  RotationMethod=None  RotationAngleUnits=deg  RotationStandardAxis=+Z  RotationAngle=0  RotationArbitraryAxis=[0 0 1]  FollAlignAxisA=+X  BaseAlignAxisA=+Y  FollAlignAxisB=+Y  BaseAlignAxisB=+Z  RotationSequenceAxes=FollowerAxes  RotationSequence=XYX  RotationSequenceAngles=[0 0 0]  RotationSequenceAnglesUnits=deg  RotationMatrix=[1 0 0; 0 1 0; 0 0 1]
  ref : PMIOPort  Side=Left
  rot : PMIOPort  Port=2  Side=Right
  angle : Outport
  wires:
  Converter3/1 -> angle/1
  connections:
  Revolute Joint/LConn1 -- Ref Rotation/RConn1
  rot/RConn1 -- Revolute Joint/RConn1
  Rigid Transform1/RConn1 -- Pos Flange/RConn1
  Rigid Transform/RConn1 -- Neg Flange/RConn1
  ref/RConn1 -- Reference Frame/RConn1 -- Ref Rotation/LConn1 -- Rigid Transform/LConn1 -- Rigid Transform1/LConn1
  Converter3/LConn1 -- Revolute Joint/RConn2
